simulink model "Etapa_2_Parte_Branca"  (R2022b)
settings: Solver=VariableStepAuto  StartTime=0.0  StopTime=20  RelTol=1e-3
settings Model: Creator=salio  LastModifiedBy=Bárbara Francisco
settings SolverCC: MaxConsecutiveMinStep=10  ZeroCrossAlgorithm=Adaptive
settings DebuggingCC: SignalInfNanChecking=error  IgnoredZcDiagnostic=none

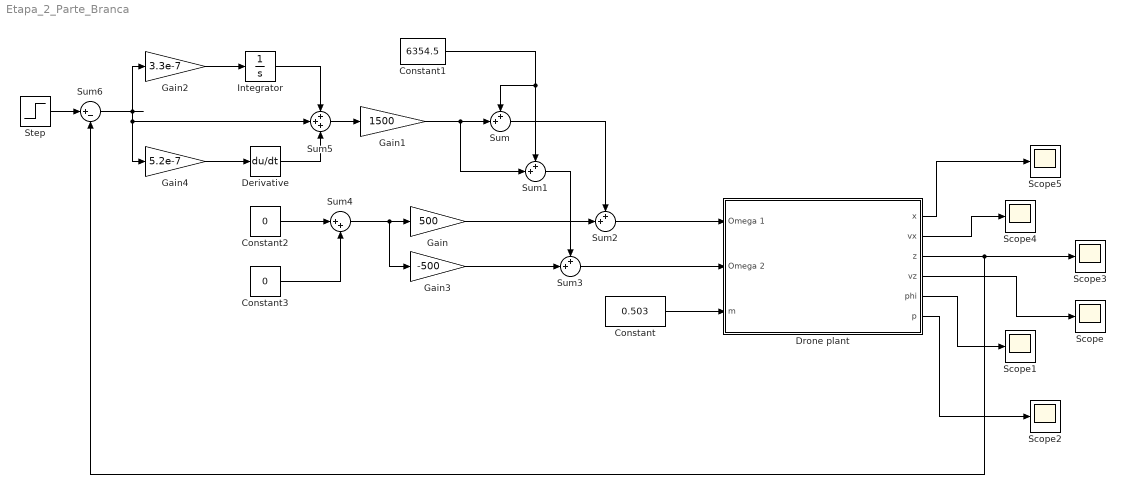
== system Etapa_2_Parte_Branca ==
  Constant : Constant  Value=0.503
  Constant1 : Constant  Value=6354.5
  Constant2 : Constant  Value=0
  Constant3 : Constant  Value=0
  Derivative : Derivative
  Drone plant : Subsystem
  Gain : Gain  Gain=500
  Gain1 : Gain  Gain=1500
  Gain2 : Gain  Gain=3.3e-7
  Gain3 : Gain  Gain=-500
  Gain4 : Gain  Gain=5.2e-7
  Integrator : Integrator
  Scope{,1..5} (6 alike) : Scope
  Step : Step  After=5  SampleTime=0
  Sum{,1..3} (4 alike) : Sum  Inputs=++|
  Sum4 : Sum  Inputs=|++
  Sum5 : Sum  Inputs=+++
  Sum6 : Sum  Inputs=|+-
  wires:
  Sum3/1 -> Drone plant/2(Omega 2)
  Constant/1 -> Drone plant/3(m)
  Drone plant/1(x) -> Scope5/1
  Drone plant/2(vx) -> Scope4/1
  Drone plant/5(phi) -> Scope1/1
  Drone plant/6(p) -> Scope2/1
  Drone plant/3(z) -> Scope3/1, Sum6/2
  Drone plant/4(vz) -> Scope/1
  Sum2/1 -> Drone plant/1(Omega 1)
  Constant1/1 -> Sum1/1, Sum/1
  Gain1/1 -> Sum1/2, Sum/2
  Sum/1 -> Sum2/1
  Gain/1 -> Sum2/2
  Sum1/1 -> Sum3/1
  Gain3/1 -> Sum3/2
  Sum4/1 -> Gain3/1, Gain/1
  Constant2/1 -> Sum4/1
  Constant3/1 -> Sum4/2
  Sum5/1 -> Gain1/1
  Integrator/1 -> Sum5/1
  Gain2/1 -> Integrator/1
  Gain4/1 -> Derivative/1
  Derivative/1 -> Sum5/3
  Sum6/1 -> Gain4/1, Sum5/2, Gain2/1
  Step/1 -> Sum6/1

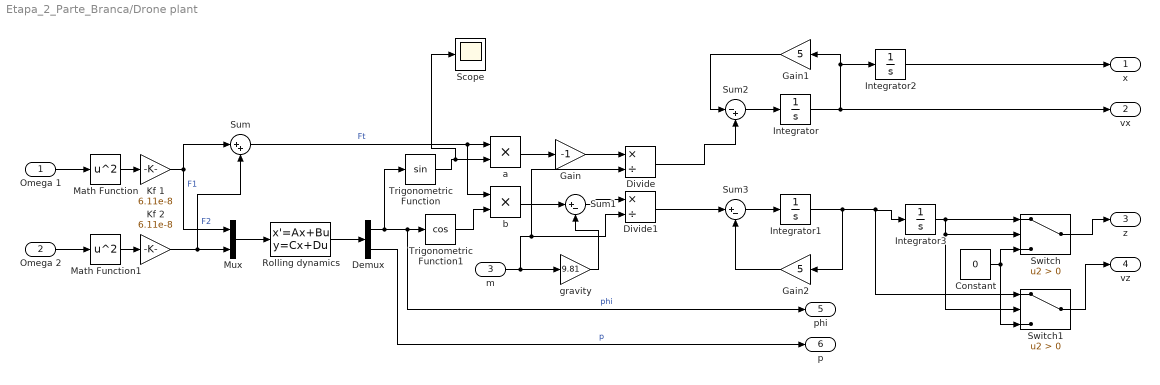
== system Etapa_2_Parte_Branca/Drone plant ==
  Omega 1 : Inport
  Omega 2 : Inport  Port=2
  m : Inport  Port=3
  Constant : Constant  Value=0
  Demux : Demux  Outputs=2
  Divide : Product  Inputs=*/
  Divide1 : Product  Inputs=*/
  Gain : Gain  Gain=-1
  Gain1 : Gain  Gain=5
  Gain2 : Gain  Gain=5
  Integrator{,1..3} (4 alike) : Integrator
  Kf 1 : Gain  Gain=6.11e-8
  Kf 2 : Gain  Gain=6.11e-8
  Math Function : Math  Operator=square
  Math Function1 : Math  Operator=square
  Mux : Mux  Inputs=2
  Rolling dynamics : StateSpace  A=[0 1; 0 -1800]  B=[0 0; 110.8 -110.8]  C=[1 0; 0 1]  D=[0 0; 0 0]  InitialCondition=0
  Scope : Scope
  Sum : Sum  Inputs=|++
  Sum1 : Sum  Inputs=|+-
  Sum2 : Sum  Inputs=|-+
  Sum3 : Sum  Inputs=|+-
  Switch : Switch  Criteria=u2 > Threshold  SaturateOnIntegerOverflow=off  InputSameDT=off
  Switch1 : Switch  Criteria=u2 > Threshold  SaturateOnIntegerOverflow=off  InputSameDT=off
  Trigonometric Function : Trigonometry
  Trigonometric Function1 : Trigonometry  Operator=cos
  a : Product
  b : Product
  gravity : Gain  Gain=9.81
  x : Outport
  vx : Outport  Port=2
  z : Outport  Port=3
  vz : Outport  Port=4
  phi : Outport  Port=5
  p : Outport  Port=6
  wires:
  Demux/1 -> phi/1, Trigonometric Function1/1, Trigonometric Function/1  "phi"
  Omega 2/1 -> Math Function1/1
  Kf 2/1 -> Mux/2, Sum/2  "F2"
  Kf 1/1 -> Mux/1, Sum/1  "F1"
  Demux/2 -> p/1  "p"
  Trigonometric Function/1 -> Scope/1, a/2
  Math Function/1 -> Kf 1/1
  Omega 1/1 -> Math Function/1
  Mux/1 -> Rolling dynamics/1
  Rolling dynamics/1 -> Demux/1
  Sum/1 -> b/1, a/1  "Ft"
  Trigonometric Function1/1 -> b/2
  Math Function1/1 -> Kf 2/1
  Switch/1 -> z/1
  a/1 -> Gain/1
  Gain/1 -> Divide/1
  Divide/1 -> Sum2/2
  Integrator2/1 -> x/1
  Divide1/1 -> Sum3/1
  Integrator3/1 -> Switch1/2, Switch/2, Switch/1
  m/1 -> Divide1/2, Divide/2, gravity/1
  b/1 -> Sum1/1
  gravity/1 -> Sum1/2
  Sum1/1 -> Divide1/1
  Integrator/1 -> vx/1, Gain1/1, Integrator2/1
  Gain1/1 -> Sum2/1
  Sum2/1 -> Integrator/1
  Sum3/1 -> Integrator1/1
  Constant/1 -> Switch1/3, Switch/3
  Switch1/1 -> vz/1
  Integrator1/1 -> Gain2/1, Switch1/1, Integrator3/1
  Gain2/1 -> Sum3/2
